simulink model "timedRef"  (R2016a)
settings: Solver=VariableStepAuto  StartTime=0.0  StopTime=10.0  RelTol=1e-3
values from neighbouring files (symbols this model uses):
  dt = 0.15    [genKUKATrajectory.m]
  Href = Ttot    [genKUKATrajectory.m]
settings Model: Creator=localadmin  LastModifiedBy=localadmin

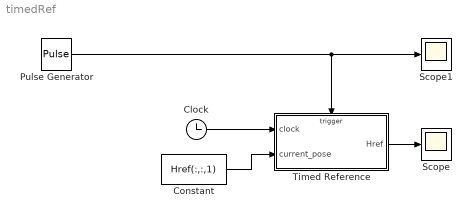
== system timedRef ==
  Clock : Clock
  Constant : Constant  Value=Href(:,:,1)
  Pulse Generator : DiscretePulseGenerator  PulseType=Time based  Period=0.1  PulseWidth=50
  Scope : Scope
  Scope1 : Scope
  Timed Reference : Subsystem  TreatAsAtomicUnit=on
  wires:
  Constant/1 -> Timed Reference/2(current_pose)
  Timed Reference/1(Href) -> Scope/1
  Clock/1 -> Timed Reference/1(clock)
  Pulse Generator/1 -> Timed Reference/Trigger, Scope1/1

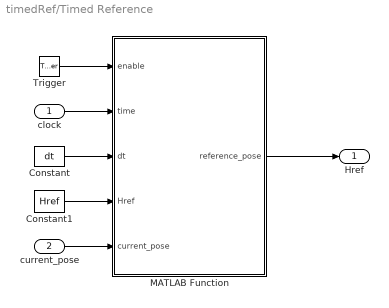
== system timedRef/Timed Reference ==
  clock : Inport
  current_pose : Inport  Port=2
  Trigger : TriggerPort  VariantControl=Variant  ShowOutputPort=on  PortDimensions=1
  Constant : Constant  Value=dt
  Constant1 : Constant  Value=Href
  MATLAB Function : MATLAB Function  TreatAsAtomicUnit=on
  Href : Outport
  wires:
  MATLAB Function/1(reference_pose) -> Href/1
  Trigger/1 -> MATLAB Function/1(enable)
  clock/1 -> MATLAB Function/2(time)
  current_pose/1 -> MATLAB Function/5(current_pose)
  Constant/1 -> MATLAB Function/3(dt)
  Constant1/1 -> MATLAB Function/4(Href)

== matlab function timedRef/Timed Reference/MATLAB Function ==
  data: enable input; reference_pose output; time input; dt input; Href input; current_pose input
function reference_pose = startReference(enable, time, dt, Href, current_pose)
% Timed output of the reference homogeneous transform. 
% Monitors a trigger send by the scheduling script to synchronize the
% command reference.
persistent startTime;
if isempty(startTime)
    startTime = 0;
end

reference_pose = current_pose;

if enable && startTime==0
    startTime = time;
end

if enable
    current_time = (time - startTime)/dt;
    reference_pose = Href(:,:,floor(current_time)+1);
end
    
end
